simulink model "KUKA_LBR_Simulink_model_flatness_based_control"  (R2017a)
settings: Solver=VariableStepAuto  StartTime=0.0  StopTime=T  RelTol=1e-3
InitFcn:
  | main
values from neighbouring files (symbols this model uses):
  elbowAngle = elbowAngle * pi/180    (= 0)    [KUKA_LBR_init.m]    (also in Untitled2.m)
  KAnaJacNum = [k_ind 0 0 0 0 0 ;                 0  k_ind 0 0 0 0 ;                    0 0 k_ind 0 0 0 ;                      0 0 0 k_ind 0 0 ;                        0 0 0 0 k_ind 0 ;                          0 0 0 0 0 k_ind ;                            ]    [KUKA_LBR_init.m]
  Kuka_LBR_param_simu = Simulink.Parameter(Kuka_LBR_param_simu)    [KUKA_LBR_init.m]
  KUKA_LBR_x0 = [x1_0 x2_0 x3_0 x4_0 x5_0 x6_0 x7_0 x8_0 x9_0 x10_0 x11_0 x12_0 x13_0 x14_0]    [KUKA_LBR_init.m]
  rpyDes = rpyDes * pi/180    [KUKA_LBR_init.m]    (also in Untitled2.m)
  T = 0.5    [KUKA_LBR_init.m]
  vecGlobalConfig = [1; 1; 1]    [KUKA_LBR_init.m]    (also in Untitled2.m = [1, 1, 1])
undefined symbols (not defined in the file or in its folder): Kuka_LBR_param
(part 4 of 19)

== matlab function KUKA_LBR_Simulink_model_flatness_based_control/KUKA_LBR_iiwa_inverse_kinematic ==
  data: vecPosDes_ input; vecJointPos output; quatOriDes_ input; jointsNum_ input; KUKA_LBR_param_ input; ellbowAngle_ input; vecGlobalConfig_ input
function vecJointPos  = KUKA_LBR_iiwa_inverse_kinematic(vecPosDes_,quatOriDes_,jointsNum_,KUKA_LBR_param_,ellbowAngle_,vecGlobalConfig_)

 
%  * Creation of a new function that calculates the jointAngles of the robot arm
%  * The function works with three variables which are necessary for calculation
%  * vecJointPos describes the current state of the jointAngles
%  * vecPosDes describes the desired state of the jointAngles
%  quatOriDes describes the desired orientation of the tool as a quaternion
%  

% set Global configuration parameters
if vecGlobalConfig_(1,1) > 0 
    lefty = 1;
else 
    lefty = -1;
end

if vecGlobalConfig_(2,1) > 0 
    ellbowUp = 1;
else 
    ellbowUp = -1;
end

if vecGlobalConfig_(3,1) > 0 
    wristIn = 1;
else 
    wristIn = -1;
end


vecJointPos = [1,1,1,1,1,1,1];

qw = quatOriDes_(1);
qx = quatOriDes_(2);
qy = quatOriDes_(3);
qz = quatOriDes_(4);

rotMatDes = [1-2*qy^2-2*qz^2, 2*qx*qy-2*qz*qw, 2*qx*qz+2*qy*qw; ...
             2*qx*qy+2*qz*qw, 1-2*qx^2-2*qz^2, 2*qy*qz-2*qx*qw; ...
             2*qx*qz-2*qy*qw, 2*qy*qz+2*qx*qw, 1-2*qx^2-2*qy^2];
         

limitsUpper = zeros(7,1);
limitsLower = zeros(7,1);

% Setting upper and lower limits for different joints
limitsUpper(1,1) = KUKA_LBR_param_.dblJoint1PosMax;
limitsUpper(2,1) = KUKA_LBR_param_.dblJoint2PosMax;
limitsUpper(3,1) = KUKA_LBR_param_.dblJoint3PosMax;
limitsUpper(4,1) = KUKA_LBR_param_.dblJoint4PosMax;
limitsUpper(5,1) = KUKA_LBR_param_.dblJoint5PosMax;
limitsUpper(6,1) = KUKA_LBR_param_.dblJoint6PosMax;
limitsUpper(7,1) = KUKA_LBR_param_.dblJoint7PosMax;

limitsLower(1,1) = KUKA_LBR_param_.dblJoint1PosMin;
limitsLower(2,1) = KUKA_LBR_param_.dblJoint2PosMin;
limitsLower(3,1) = KUKA_LBR_param_.dblJoint3PosMin;
limitsLower(4,1) = KUKA_LBR_param_.dblJoint4PosMin;
limitsLower(5,1) = KUKA_LBR_param_.dblJoint5PosMin;
limitsLower(6,1) = KUKA_LBR_param_.dblJoint6PosMin;
limitsLower(7,1) = KUKA_LBR_param_.dblJoint7PosMin;

%Vector from Base to shoulder
vecBasetoJoint2 = [0,0,KUKA_LBR_param_.dblLinkBase1Len]';

%Vector from Wrist to endeffector
vecJoint6to7 = [0,0,KUKA_LBR_param_.dblLink67Len]';

%vector from shoulder to wrist

vecJoint2to6 = vecPosDes_' - vecBasetoJoint2 - (rotMatDes * vecJoint6to7);

%calculate unit vector from shoulder to wrist

distJoint2To6 = norm(vecJoint2to6);

vecDirectionJoint2To6 = vecJoint2to6/distJoint2To6;

skewMatDirJoint2to6 = zeros(3,3);

skewMatDirJoint2to6(1,1) = 0;
skewMatDirJoint2to6(1,2) = -vecDirectionJoint2To6(3,1);
skewMatDirJoint2to6(1,3) = vecDirectionJoint2To6(2,1);
skewMatDirJoint2to6(2,1) = vecDirectionJoint2To6(3,1);
skewMatDirJoint2to6(2,2) = 0;
skewMatDirJoint2to6(2,3) = -vecDirectionJoint2To6(1,1);
skewMatDirJoint2to6(3,1) = -vecDirectionJoint2To6(2,1);
skewMatDirJoint2to6(3,2) = vecDirectionJoint2To6(1,1);
skewMatDirJoint2to6(3,3) = 0;

argument4 = (distJoint2To6.^2 - KUKA_LBR_param_.dblLink23Len.^2 - KUKA_LBR_param_.dblLink45Len.^2)/(2 * KUKA_LBR_param_.dblLink45Len *  KUKA_LBR_param_.dblLink23Len);

referenceAngle4 = ellbowUp * acos(checkArgument(argument4));

if (referenceAngle4 > limitsUpper(4,1) || referenceAngle4 < limitsLower(4,1) || isnan(referenceAngle4))
    error('limits of joint Angle 4 exceeded');
        

end

%calculation of help angles alpha and beta

argument_alpha = vecJoint2to6(3,1) / distJoint2To6;

alpha = asin(checkArgument(argument_alpha));

argument_beta = (KUKA_LBR_param_.dblLink23Len.^2 + distJoint2To6.^2 - KUKA_LBR_param_.dblLink45Len.^2)/( 2 * KUKA_LBR_param_.dblLink23Len * distJoint2To6);

beta = acos(checkArgument(argument_beta));

%calculation of reference Angle 1 wih alpha and beta

referenceAngle1 = atan2(vecJoint2to6(2,1),vecJoint2to6(1,1));

referenceAngle2 = pi/2 - alpha - ellbowUp * beta;

referenceAngle3 = 0;

%vecReferenceAngles = [referenceAngle1 , referenceAngle2, referenceAngle3, referenceAngle4];

IMat3x3 = eye(3);

rotMatEllbowAngle = IMat3x3 + sin(ellbowAngle_) * skewMatDirJoint2to6 + (1-cos(ellbowAngle_)) * skewMatDirJoint2to6.^2;

veclinklengths = [KUKA_LBR_param_.dblLinkBase1Len; 0; KUKA_LBR_param_.dblLink23Len; 0; KUKA_LBR_param_.dblLink45Len; 0; KUKA_LBR_param_.dblLink67Len];

vecRotbetweenJoints = [-pi/2, pi/2,pi/2,-pi/2,-pi/2,pi/2,0];

refTransMat0to1 = denavitHardenbergTransformation(vecRotbetweenJoints(1,1), veclinklengths(1), referenceAngle1);

refTransMat1to2 = denavitHardenbergTransformation(vecRotbetweenJoints(1,2), veclinklengths(2), referenceAngle2);

refTransMat2to3 = denavitHardenbergTransformation(vecRotbetweenJoints(1,3), veclinklengths(3), referenceAngle3);

refTransMat3to4 = denavitHardenbergTransformation(vecRotbetweenJoints(1,4), veclinklengths(4), referenceAngle4);

refTransMat0to3 = refTransMat0to1 + refTransMat1to2 + refTransMat2to3;

refTransMat0to4 = refTransMat0to3 + refTransMat3to4;


%Identification of the rotation matrices of the refernce syste%

refRotMat0to3 = refTransMat0to3(1:3,1:3);

refRotMat0to4 = refTransMat0to4(1:3,1:3);

coeffMatAs = skewMatDirJoint2to6 * refRotMat0to3;

coeffMatBs = - (skewMatDirJoint2to6 * skewMatDirJoint2to6) * refRotMat0to3;

coeffMatCs = (IMat3x3 + skewMatDirJoint2to6) * refRotMat0to3;

jointAngle1 = atan2(lefty * (-coeffMatAs(2,2) * sin(ellbowAngle_) ...
         - coeffMatBs(2,2) * cos(ellbowAngle_) - coeffMatCs(2,2)), ...
          lefty * (coeffMatAs(1,2) * sin(ellbowAngle_) ... 
          - coeffMatBs(1,2) * cos(ellbowAngle_) - coeffMatCs(1,2)));
      
if (jointAngle1 > limitsUpper(1,1) || jointAngle1 < limitsLower(1,1)) 
    error('Limits of joinAngle1 exceeded!');
        
end

argument2 = -coeffMatAs(3,2) * sin(ellbowAngle_) ...
            - coeffMatBs(3,2) * cos(ellbowAngle_) ...
            - coeffMatCs(3,2);
        
jointAngle2 = lefty * acos(checkArgument(argument2));

if (jointAngle2 > limitsUpper(2,1) || jointAngle2 < limitsLower(2,1))
    error('Limits of joinAngle2 exceeded!');
        
end

jointAngle3 = atan2(lefty * coeffMatAs(3,3) * sin(ellbowAngle_) ...
                    + coeffMatBs(3,3) * cos(ellbowAngle_) ...
                    + coeffMatCs(2,2), ... 
                    lefty * (-coeffMatAs(3,1) * sin(ellbowAngle_)...
                    - coeffMatBs(3,1) * cos(ellbowAngle_) ...
                    - coeffMatCs(3,1)));

if (jointAngle3 > limitsUpper(3,1) || jointAngle3 < limitsLower(3,1))
   error('Limits of joinAngle3 exceeded!');
        
end

jointAngle4 = referenceAngle4;

if (jointAngle4 > limitsUpper(4,1) || jointAngle4 < limitsLower(4,1))
    error('Limits of joinAngle4 exceeded!');
      
end

rotMat0to3 = rotMatEllbowAngle * refRotMat0to3;
rotMat0to4 = rotMatEllbowAngle * refRotMat0to4;
rotMat3to4 = transpose(rotMat0to3) * rotMat0to4;

coeffMatAw = transpose(rotMat3to4) * transpose(coeffMatAs) * rotMatDes;
coeffMatBw = transpose(rotMat3to4) * transpose(coeffMatBs) * rotMatDes;
coeffMatCw = transpose(rotMat3to4) * transpose(coeffMatCs) * rotMatDes;

%Calculation of jointAngle5 with the coefficient matrices

jointAngle5 = atan2(wristIn * coeffMatAw(2,3) * sin(ellbowAngle_) ...
              + coeffMatBw(2,3) * cos(ellbowAngle_) ... 
              + coeffMatCw(2,3), ...
              wristIn *(coeffMatAw(1,3) * sin(ellbowAngle_) ...
              + coeffMatBw(1,3) * cos(ellbowAngle_) ...
              + coeffMatCw(1,3)));


if (jointAngle5 > limitsUpper(5,1) || jointAngle5 < limitsLower(5,1))
     error('Limits of joinAngle5 exceeded!');
      
end 
    
argument6 = coeffMatAw(3,3) * sin(ellbowAngle_) ...
            + coeffMatBw(3,3) * cos(ellbowAngle_) ...
                  + coeffMatCw(3,3);

jointAngle6 = wristIn * acos(checkArgument(argument6));

if (jointAngle6 > limitsUpper(6,1) || jointAngle6 < limitsLower(6,1))
      error('Limits of joinAngle6 exceeded!');
      
end 

jointAngle7 = atan2(wristIn * (coeffMatAw(3,2) * sin(ellbowAngle_) ...
            + coeffMatBw(3,2) * cos(ellbowAngle_) ...
            + coeffMatCw(3,2)), ...
            wristIn * (-coeffMatAw(3,1) * sin(ellbowAngle_) ...
            - coeffMatBw(3,1) * cos(ellbowAngle_)...
            -coeffMatCw(3,1)));

if (jointAngle7 > limitsUpper(7,1) || jointAngle7 < limitsLower(7,1))
       error('Limits of joinAngle7 exceeded!');
        
end

    vecJointPos(1) = jointAngle1;
    vecJointPos(2) = jointAngle2;
    vecJointPos(3) = jointAngle3;
    vecJointPos(4) = -jointAngle4;
    vecJointPos(5) = jointAngle5;
    vecJointPos(6) = jointAngle6;
    vecJointPos(7) = jointAngle7;
end



function [rotmat] = denavitHardenbergTransformation(alpha_,theta_,d_)


matRot = rotx(alpha_) * rotz(theta_);

vecTrans = [0;0;d_];

matTrans = [matRot vecTrans];

rotmat = [matTrans; 0 0 0 1];

end

function [argument_] = checkArgument(argument_)

if argument_ < -1.0
    if argument_ < -1.001
        error('Invalid Argument');
        
    else
        argument_ = -1.0;
    end
elseif argument_ > 1.0
        if argument_ > 1.001
            error('Invalid Argument');
        
        end
    else
        argument_ = 1.0;

end
end


function rotxAlpha  = rotx(alpha_)
rotxAlpha = [1 0           0; ...
             0 cos(alpha_) -sin(alpha_); ... 
             0 sin(alpha_) cos(alpha_)];
end

function rotzTheta  = rotz(theta_)
rotzTheta = [cos(theta_) -sin(theta_) 0; ... 
             sin(theta_) cos(theta_)  0; ...
             0           0            1];
end
